simulink model "simulink"  (R2023a)
settings: Solver=FixedStepAuto  StartTime=0.0  StopTime=100  FixedStep=1e-3  RelTol=1e-3
undefined symbols (not defined in the file): A, B, b, B2, J, Ke, Kt, L, L_0, M, Phi, R, S, S2
settings Model: Creator=bonnin15u  LastModifiedBy=bonnin15u

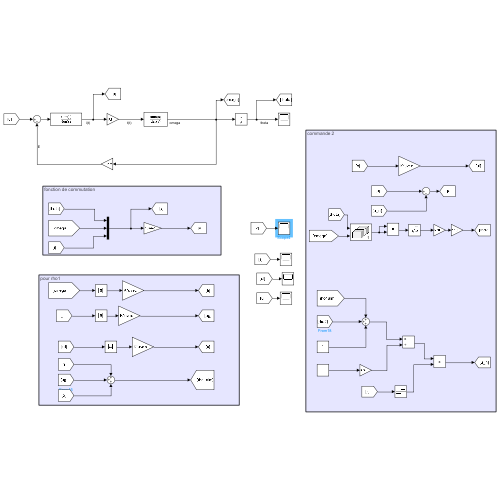
[thumbnail: Simulink's stored preview of the top-level diagram]
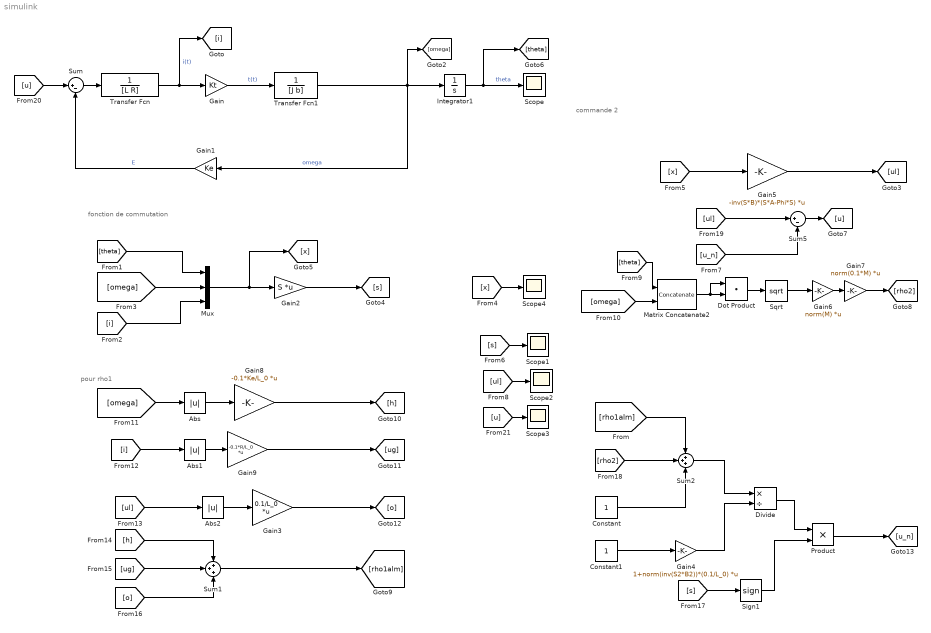
== system simulink ==
  note: pour rho1
  note: fonction de commutation
  note: commande 2
  Abs : Abs  SaturateOnIntegerOverflow=off
  Abs1 : Abs  SaturateOnIntegerOverflow=off
  Abs2 : Abs  SaturateOnIntegerOverflow=off
  Constant : Constant
  Constant1 : Constant
  Divide : Product  Inputs=*/
  Dot Product : DotProduct  OutDataTypeStr=Inherit: Inherit via internal rule
  Gain : Gain  Gain=Kt
  Gain1 : Gain  Gain=Ke
  Gain2 : Gain  Gain=S  Multiplication=Matrix(K*u) (u vector)
  Gain3 : Gain  Gain=0.1/L_0  Multiplication=Matrix(K*u) (u vector)
  Gain4 : Gain  Gain=1+norm(inv(S2*B2))*(0.1/L_0)  Multiplication=Matrix(K*u)
  Gain5 : Gain  Gain=-inv(S*B)*(S*A-Phi*S)  Multiplication=Matrix(K*u) (u vector)
  Gain6 : Gain  Gain=norm(M)  Multiplication=Matrix(K*u)
  Gain7 : Gain  Gain=norm(0.1*M)  Multiplication=Matrix(K*u)
  Gain8 : Gain  Gain=-0.1*Ke/L_0  Multiplication=Matrix(K*u) (u vector)
  Gain9 : Gain  Gain=-0.1*R/L_0  Multiplication=Matrix(K*u) (u vector)
  Integrator1 : Integrator  InitialCondition=3
  Matrix Concatenate2 : Concatenate  Mode=Multidimensional array
  Mux : Mux  Inputs=3
  Product : Product
  Scope{,1..4} (5 alike) : Scope
  Sign1 : Signum
  Sqrt : Sqrt
  Sum : Sum  Inputs=|+-
  Sum1 : Sum  Inputs=+++
  Sum2 : Sum  Inputs=+++
  Sum5 : Sum  Inputs=|+-
  Transfer Fcn : TransferFcn  Denominator=[L R]
  Transfer Fcn1 : TransferFcn  Denominator=[J b]
  wires:
  Gain1/1 -> Sum/2  "E"
  Sum/1 -> Transfer Fcn/1
  Transfer Fcn1/1 -> [omega], Integrator1/1, Gain1/1  "omega"
  Transfer Fcn/1 -> [i], Gain/1  "i(t)"
  Gain/1 -> Transfer Fcn1/1  "t(t)"
  Gain2/1 -> [s]
  [theta] -> Mux/1
  [i] -> Mux/3
  [omega] -> Mux/2
  Mux/1 -> [x], Gain2/1
  Gain5/1 -> [ul]
  [x] -> Gain5/1
  [s] -> Scope1/1
  [ul] -> Scope2/1
  Integrator1/1 -> [theta], Scope/1  "theta"
  Sqrt/1 -> Gain6/1
  Gain6/1 -> Gain7/1
  Gain7/1 -> [rho2]
  Dot Product/1 -> Sqrt/1
  [omega] -> Abs/1
  Gain8/1 -> [h]
  [i] -> Abs1/1
  Gain9/1 -> [ug]
  [ul] -> Abs2/1
  Abs2/1 -> Gain3/1
  [ug] -> Sum1/2
  [h] -> Sum1/1
  Sign1/1 -> Product/2
  [s] -> Sign1/1
  [rho1alm] -> Sum2/1
  [rho2] -> Sum2/2
  Product/1 -> [u_n]
  Sum5/1 -> [u]
  [ul] -> Sum5/1
  [theta] -> Matrix Concatenate2/1
  [omega] -> Matrix Concatenate2/2
  Matrix Concatenate2/1 -> Dot Product/1, Dot Product/2
  Constant/1 -> Sum2/3
  [u] -> Scope3/1
  [o] -> Sum1/3
  Abs/1 -> Gain8/1
  Abs1/1 -> Gain9/1
  Gain3/1 -> [o]
  Sum1/1 -> [rho1alm]
  Sum2/1 -> Divide/1
  Gain4/1 -> Divide/2
  Constant1/1 -> Gain4/1
  Divide/1 -> Product/1
  [x] -> Scope4/1
  [u] -> Sum/1
  [u_n] -> Sum5/2
